simulink model "Blocks_Basic"  (R2023a)
settings: Solver=VariableStepAuto  StartTime=0.0  StopTime=10.0  RelTol=1e-3
settings Model: Creator=SAINATH  LastModifiedBy=SAINATH

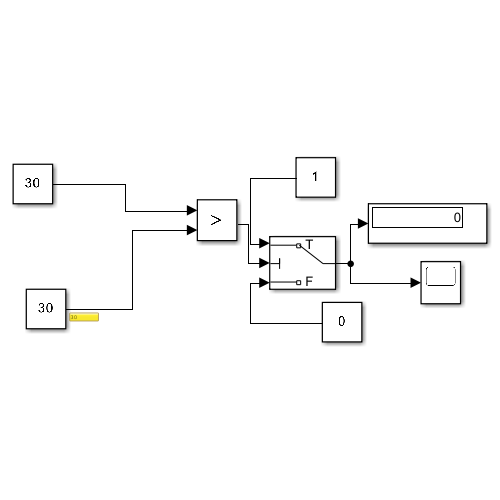
[thumbnail: Simulink's stored preview of the top-level diagram]
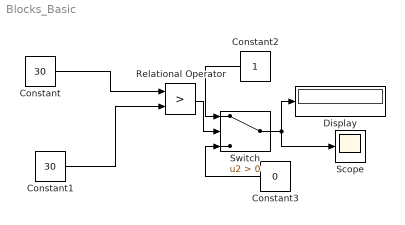
== system Blocks_Basic ==
  Constant : Constant  Value=30
  Constant1 : Constant  Value=30
  Constant2 : Constant
  Constant3 : Constant  Value=0
  Display : Display
  Relational Operator : RelationalOperator  Operator=>  OutDataTypeStr=boolean  RndMeth=Simplest  InputSameDT=off
  Scope : Scope
  Switch : Switch  Criteria=u2 > Threshold  SaturateOnIntegerOverflow=off  InputSameDT=off
  wires:
  Constant/1 -> Relational Operator/1
  Constant1/1 -> Relational Operator/2
  Relational Operator/1 -> Switch/2
  Constant2/1 -> Switch/1
  Constant3/1 -> Switch/3
  Switch/1 -> Display/1, Scope/1
